simulink model "Zadanie_3_4_5"  (R2023b)
settings: Solver=VariableStepAuto  StartTime=0.0  StopTime=10  RelTol=1e-3
undefined symbols (not defined in the file or in its folder): m, R, v_phi, v_q, x0, y0
libraries: slpidlib x2
settings Model: Creator=student  LastModifiedBy=lukin

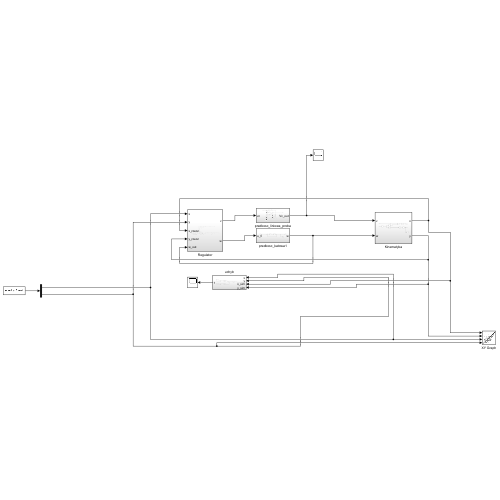
[thumbnail: Simulink's stored preview of the top-level diagram]
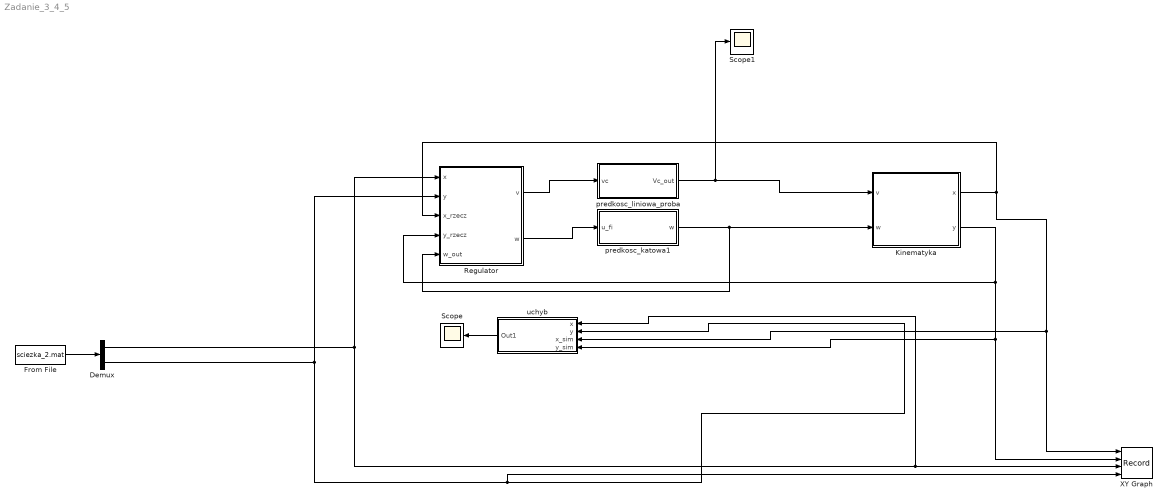
== system Zadanie_3_4_5 ==
  Demux : Demux  Outputs=2
  From File : FromFile  FileName=sciezka_2.mat  SampleTime=0
  Kinematyka : Subsystem
  Regulator : Subsystem
  Scope : Scope
  Scope1 : Scope
  XY Graph : Record  FileSettingsInternal="{\"entries\":[{\"content\":{\"excelSettings\":{\"content\":{},\"type\":\"Streamout.ExcelSettings\"}},\"type\":\"Streamout.FileSettingStorage\",\"uuid\":\"\"}],\"packageUris\":[\"http:\\/\\/schema.mathworks.com\\/mf0\\/streamout_blocks\\/R2020a\"],\"version\":\"1.0\"}"  Layout=[1 1]  SignalsInternal="{\"entries\":[{\"content\":{\"signals\":[{\"content\":{\"blockPath\":[],\"dimensions\":[1],\"domain\":\"\",\"lineColor\":\"#edb120\",\"plots\":[ 1 ],\"port\":1,\"sid\":[\"\"],\"signalID\":1,\"signalName\":\"Kinematyka:1\"},\"type\":\"RecordBlkView.Signal\",\"uuid\":\"\"},{\"content\":{\"blockPath\":[],\"dimensions\":[1],\"domain\":\"\",\"lineColor\":\"#7e2f8e\",\"plots\":[ 1 ],\"port\":2,\"sid\":[\"\"],\"signalID\":2,\"signalName\":\"Kinematyka:2\"},\"type\":\"RecordBlkView.Signal\",\"uuid\":\"\"},{\"content\":{\"blockPath\":[],\"dimensions\":[1],\"domain\":\"\",\"lineColor\":\"#7e2f8e\",\"plots\":[ 1 ],\"port\":3,\"sid\":[\"\"],\"signalID\":3,\"signalName\":\"Demux:1\"},\"type\":\"RecordBlkView.Signal\",\"uuid\":\"\"},{\"content\":{\"blockPath\":[],\"dimensions\":[1],\"domain\":\"\",\"lineColor\":\"#77ac30\",\"plots\":[ 1 ],\"port\":4,\"sid\":[\"\"],\"signalID\":4,\"signalName\":\"Demux:2\"},\"type\":\"RecordBlkView.Signal\",\"uuid\":\"\"}]},\"type\":\"RecordBlkView.InputSignals\",\"uuid\":\"\"}],\"packageUris\":[\"http:\\/\\/schema.mathworks.com\\/mf0\\/streamout_blocks\\/R2020a\"],\"version\":\"1.0\"}"  VisualizationBindings="{\"xyplotplugin\":{\"info\":[{\"series\":[{\"bindingParametersList\":[{\"parameter\":\"X-Axis\",\"signalID\":1,\"signalName\":\"Kinematyka:1\"},{\"parameter\":\"Y-Axis\",\"signalID\":2,\"signalName\":\"Kinematyka:2\"}],\"seriesID\":0},{\"bindingParametersList\":[{\"parameter\":\"X-Axis\",\"signalID\":3,\"signalName\":\"Demux:1\"},{\"parameter\":\"Y-Axis\",\"signalID\":4,\"signalName\":\"Demux:2\"}],\"seriesID\":1},{\"bindingParametersList\":[{\"parameter\":\"Y-Axis\",\"signalID\":4,\"signalName\":\"Demux:2\"}],\"seriesID\":2}],\"subplotID\":1}]}}"  CompatibilityTag=XY  st=-1
  predkosc_katowa1 : Subsystem
  predkosc_liniowa_proba : Subsystem
  uchyb : Subsystem
  wires:
  From File/1 -> Demux/1
  Demux/1 -> XY Graph/3, uchyb/1(x), Regulator/1(x)
  Demux/2 -> XY Graph/4, uchyb/2(y), Regulator/2(y)
  Kinematyka/1(x) -> XY Graph/1, uchyb/3(x_sim), Regulator/3(x_rzecz)
  Kinematyka/2(y) -> XY Graph/2, uchyb/4(y_sim), Regulator/4(y_rzecz)
  uchyb/1(Out1) -> Scope/1
  Regulator/2(w) -> predkosc_katowa1/1(u_fi)
  predkosc_katowa1/1(w) -> Regulator/5(w_out), Kinematyka/2(w)
  Regulator/1(v) -> predkosc_liniowa_proba/1(vc)
  predkosc_liniowa_proba/1(Vc_out) -> Kinematyka/1(v), Scope1/1

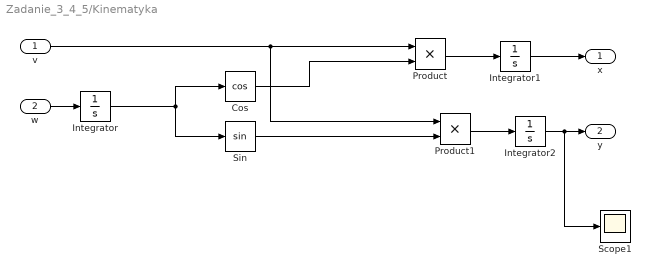
== system Zadanie_3_4_5/Kinematyka ==
  v : Inport
  w : Inport  Port=2
  Cos : Trigonometry  Operator=cos
  Integrator : Integrator  InitialCondition=v_phi
  Integrator1 : Integrator  InitialCondition=x0
  Integrator2 : Integrator  InitialCondition=y0
  Product : Product
  Product1 : Product
  Scope1 : Scope
  Sin : Trigonometry
  x : Outport
  y : Outport  Port=2
  wires:
  v/1 -> Product1/1, Product/1
  Cos/1 -> Product/2
  Product/1 -> Integrator1/1
  Integrator1/1 -> x/1
  Sin/1 -> Product1/2
  Product1/1 -> Integrator2/1
  Integrator2/1 -> Scope1/1, y/1
  w/1 -> Integrator/1
  Integrator/1 -> Cos/1, Sin/1

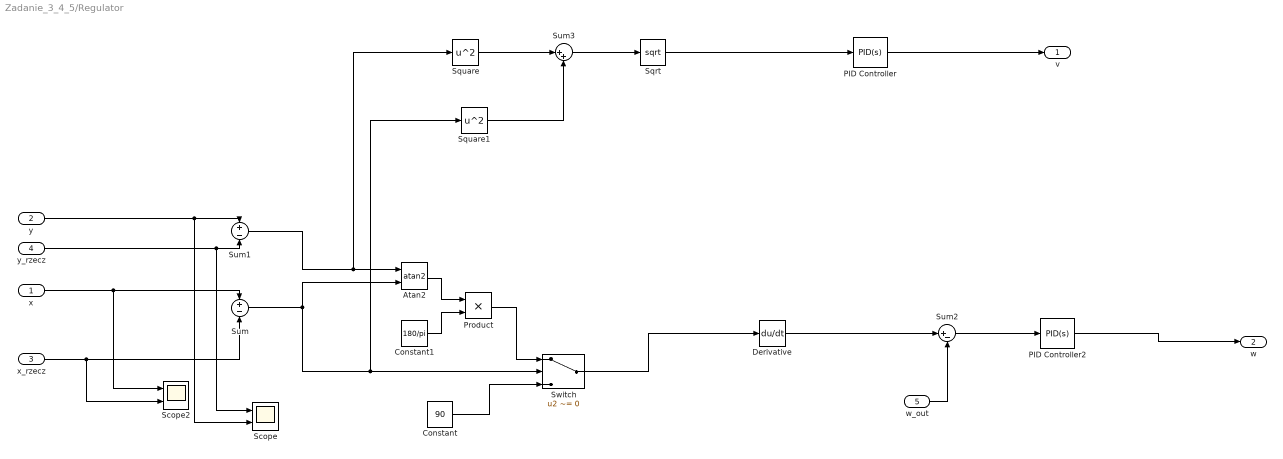
== system Zadanie_3_4_5/Regulator ==
  x : Inport
  y : Inport  Port=2
  x_rzecz : Inport  Port=3
  y_rzecz : Inport  Port=4
  w_out : Inport  Port=5
  Atan2 : Trigonometry  Operator=atan2  OutputSignalType=real
  Constant : Constant  Value=90
  Constant1 : Constant  Value=180/pi
  Derivative : Derivative
  PID Controller : slpidlib/PID Controller  Controller=PID  Form=Parallel  TimeDomain=Continuous-time  UseExternalTs=off  SampleTime=-1  IntegratorMethod=Forward Euler  FilterMethod=Forward Euler  ControllerParametersSource=internal  P=1.8  I=0  UseKiTs=off  D=0  N=100  UseFilter=on  TunerSelectOption=Transfer Function Based (PID Tuner App)  InitialConditionSource=internal  InitialConditionForIntegrator=0  InitialConditionForFilter=0  DifferentiatorICPrevScaledInput=0  ExternalReset=none  TrackingMode=off  Kt=1  LimitOutput=off  SatLimitsSource=internal  UpperSaturationLimit=inf  LowerSaturationLimit=-inf  LinearizeAsGain=on  AntiWindupMode=none  Kb=1  LimitIntegrator=off  UpperIntegratorSaturationLimit=inf  LowerIntegratorSaturationLimit=-inf  POutMin=[]  POutMax=[]  IOutMin=[]  IOutMax=[]  DOutMin=[]  DOutMax=[]  NOutMin=[]  NOutMax=[]  SumOutMin=[]  SumOutMax=[]  SaturationOutMin=[]  SaturationOutMax=[]  PParamMin=[]  PParamMax=[]  IParamMin=[]  IParamMax=[]  DParamMin=[]  DParamMax=[]  NParamMin=[]  NParamMax=[]  KbParamMin=[]  KbParamMax=[]  KtParamMin=[]  KtParamMax=[]  KbOutMin=[]  KbOutMax=[]  KtOutMin=[]  KtOutMax=[]  IntegratorOutMin=[]  IntegratorOutMax=[]  FilterOutMin=[]  FilterOutMax=[]  SumI1OutMin=[]  SumI1OutMax=[]  SumI2OutMin=[]  SumI2OutMax=[]  SumI3OutMin=[]  SumI3OutMax=[]  SumI4OutMin=[]  SumI4OutMax=[]  SumDOutMin=[]  SumDOutMax=[]  DifferentiatorOutMin=[]  DifferentiatorOutMax=[]  FilterDiffOutCoefMin=[]  FilterDiffOutCoefMax=[]  ReciprocalOutMin=[]  ReciprocalOutMax=[]  SumDenOutMin=[]  SumDenOutMax=[]  SumNumOutMin=[]  SumNumOutMax=[]  DivideOutMin=[]  DivideOutMax=[]  UdiffTsProdOutMin=[]  UdiffTsProdOutMax=[]  NTsProdOutMin=[]  NTsProdOutMax=[]  UintegralTsProdOutMin=[]  UintegralTsProdOutMax=[]  UngainTsProdOutMin=[]  UngainTsProdOutMax=[]  ClampingZeroOutDataTypeStr=Inherit: Inherit via back propagation  ClampingZeroOutMin=[]  ClampingZeroOutMax=[]  FilterDenConstantOutDataTypeStr=Inherit: Inherit via back propagation  FilterDenConstantOutMin=[]  FilterDenConstantOutMax=[]  PCopyOutDataTypeStr=Inherit: Inherit via back propagation  PCopyOutMin=[]  PCopyOutMax=[]  NCopyOutDataTypeStr=Inherit: Inherit via back propagation  NCopyOutMin=[]  NCopyOutMax=[]  IntegratorContinuousStateAttributes=''  IntegratorStateMustResolveToSignalObject=off  IntegratorRTWStateStorageClass=Auto  FilterContinuousStateAttributes=''  FilterStateMustResolveToSignalObject=off  FilterRTWStateStorageClass=Auto  ParallelPVariant=InternalParameters  IdealPVariant=Disabled  IVariant=InternalParameters  DVariant=InternalParameters  IntegratorVariant=Continuous  SatVariant=Disabled  AWVariant=Passthrough  PCopyVariant=Disabled  TRVariant=Disabled  FdbkBlocksVariant=Forward  IdealPFdbkVariant=Disabled  SatFdbkVariant=Disabled  DerivativeFilterVariant=ContFilter  NVariant=InternalParameters  NCopyVariant=Disabled  FilterICVariant=InternalICsFilter  IntegratorICVariant=InternalICs  ExternalResetVariant=Disabled  TRSumVariant=Passthrough  SumFdbkVariant=Disabled  SumVariant=Sum_PID  TsampFilterVariant=InternalTs  TsampNgainVariant=Passthrough  TsampIntegralVariant=Disabled_SignalSpec  ExternalSaturationOutDataTypeStr=Inherit: Same as second input
  PID Controller2 : slpidlib/PID Controller  Controller=PID  Form=Parallel  TimeDomain=Continuous-time  UseExternalTs=off  SampleTime=-1  IntegratorMethod=Forward Euler  FilterMethod=Forward Euler  ControllerParametersSource=internal  P=0.65  I=0.012  UseKiTs=off  D=0.012  N=100  UseFilter=on  TunerSelectOption=Transfer Function Based (PID Tuner App)  InitialConditionSource=internal  InitialConditionForIntegrator=0  InitialConditionForFilter=0  DifferentiatorICPrevScaledInput=0  ExternalReset=none  TrackingMode=off  Kt=1  LimitOutput=off  SatLimitsSource=internal  UpperSaturationLimit=inf  LowerSaturationLimit=-inf  LinearizeAsGain=on  AntiWindupMode=none  Kb=1  LimitIntegrator=off  UpperIntegratorSaturationLimit=inf  LowerIntegratorSaturationLimit=-inf  POutMin=[]  POutMax=[]  IOutMin=[]  IOutMax=[]  DOutMin=[]  DOutMax=[]  NOutMin=[]  NOutMax=[]  SumOutMin=[]  SumOutMax=[]  SaturationOutMin=[]  SaturationOutMax=[]  PParamMin=[]  PParamMax=[]  IParamMin=[]  IParamMax=[]  DParamMin=[]  DParamMax=[]  NParamMin=[]  NParamMax=[]  KbParamMin=[]  KbParamMax=[]  KtParamMin=[]  KtParamMax=[]  KbOutMin=[]  KbOutMax=[]  KtOutMin=[]  KtOutMax=[]  IntegratorOutMin=[]  IntegratorOutMax=[]  FilterOutMin=[]  FilterOutMax=[]  SumI1OutMin=[]  SumI1OutMax=[]  SumI2OutMin=[]  SumI2OutMax=[]  SumI3OutMin=[]  SumI3OutMax=[]  SumI4OutMin=[]  SumI4OutMax=[]  SumDOutMin=[]  SumDOutMax=[]  DifferentiatorOutMin=[]  DifferentiatorOutMax=[]  FilterDiffOutCoefMin=[]  FilterDiffOutCoefMax=[]  ReciprocalOutMin=[]  ReciprocalOutMax=[]  SumDenOutMin=[]  SumDenOutMax=[]  SumNumOutMin=[]  SumNumOutMax=[]  DivideOutMin=[]  DivideOutMax=[]  UdiffTsProdOutMin=[]  UdiffTsProdOutMax=[]  NTsProdOutMin=[]  NTsProdOutMax=[]  UintegralTsProdOutMin=[]  UintegralTsProdOutMax=[]  UngainTsProdOutMin=[]  UngainTsProdOutMax=[]  ClampingZeroOutDataTypeStr=Inherit: Inherit via back propagation  ClampingZeroOutMin=[]  ClampingZeroOutMax=[]  FilterDenConstantOutDataTypeStr=Inherit: Inherit via back propagation  FilterDenConstantOutMin=[]  FilterDenConstantOutMax=[]  PCopyOutDataTypeStr=Inherit: Inherit via back propagation  PCopyOutMin=[]  PCopyOutMax=[]  NCopyOutDataTypeStr=Inherit: Inherit via back propagation  NCopyOutMin=[]  NCopyOutMax=[]  IntegratorContinuousStateAttributes=''  IntegratorStateMustResolveToSignalObject=off  IntegratorRTWStateStorageClass=Auto  FilterContinuousStateAttributes=''  FilterStateMustResolveToSignalObject=off  FilterRTWStateStorageClass=Auto  ParallelPVariant=InternalParameters  IdealPVariant=Disabled  IVariant=InternalParameters  DVariant=InternalParameters  IntegratorVariant=Continuous  SatVariant=Disabled  AWVariant=Passthrough  PCopyVariant=Disabled  TRVariant=Disabled  FdbkBlocksVariant=Forward  IdealPFdbkVariant=Disabled  SatFdbkVariant=Disabled  DerivativeFilterVariant=ContFilter  NVariant=InternalParameters  NCopyVariant=Disabled  FilterICVariant=InternalICsFilter  IntegratorICVariant=InternalICs  ExternalResetVariant=Disabled  TRSumVariant=Passthrough  SumFdbkVariant=Disabled  SumVariant=Sum_PID  TsampFilterVariant=InternalTs  TsampNgainVariant=Passthrough  TsampIntegralVariant=Disabled_SignalSpec  ExternalSaturationOutDataTypeStr=Inherit: Same as second input
  Product : Product
  Scope : Scope  NumInputPorts=2
  Scope2 : Scope  NumInputPorts=2
  Sqrt : Sqrt
  Square : Math  Operator=square
  Square1 : Math  Operator=square
  Sum : Sum  Inputs=+-
  Sum1 : Sum  Inputs=+-
  Sum2 : Sum  Inputs=|+-
  Sum3 : Sum  Inputs=|++
  Switch : Switch  Criteria=u2 ~= 0  SaturateOnIntegerOverflow=off  InputSameDT=off
  v : Outport
  w : Outport  Port=2
  wires:
  x/1 -> Scope2/1, Sum/1
  Atan2/1 -> Product/1
  Constant1/1 -> Product/2
  x_rzecz/1 -> Scope2/2, Sum/2
  y_rzecz/1 -> Scope/1, Sum1/2
  Sum2/1 -> PID Controller2/1
  w_out/1 -> Sum2/2
  Switch/1 -> Derivative/1
  Constant/1 -> Switch/3
  Product/1 -> Switch/1
  Sum1/1 -> Square/1, Atan2/1
  Sum/1 -> Square1/1, Switch/2, Atan2/2
  Derivative/1 -> Sum2/1
  y/1 -> Scope/2, Sum1/1
  Square/1 -> Sum3/1
  Square1/1 -> Sum3/2
  Sum3/1 -> Sqrt/1
  PID Controller2/1 -> w/1
  Sqrt/1 -> PID Controller/1
  PID Controller/1 -> v/1

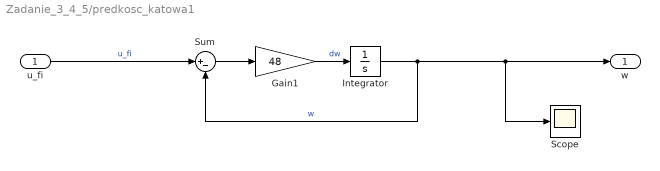
== system Zadanie_3_4_5/predkosc_katowa1 ==
  u_fi : Inport
  Gain1 : Gain  Gain=48
  Integrator : Integrator
  Scope : Scope
  Sum : Sum  Inputs=|+-
  w : Outport
  wires:
  Sum/1 -> Gain1/1
  u_fi/1 -> Sum/1  "u_fi"
  Integrator/1 -> w/1, Scope/1, Sum/2  "w"
  Gain1/1 -> Integrator/1  "dw"

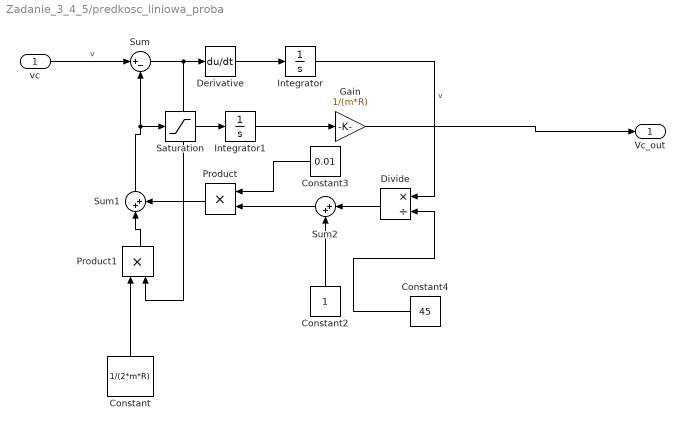
== system Zadanie_3_4_5/predkosc_liniowa_proba ==
  vc : Inport
  Constant : Constant  Value=1/(2*m*R)
  Constant2 : Constant
  Constant3 : Constant  Value=0.01
  Constant4 : Constant  Value=45
  Derivative : Derivative
  Divide : Product  Inputs=*/
  Gain : Gain  Gain=1/(m*R)
  Integrator : Integrator
  Integrator1 : Integrator  InitialCondition=v_q
  Product : Product
  Product1 : Product
  Saturation : Saturate  UpperLimit=10  LowerLimit=-10
  Sum : Sum  Inputs=|+-
  Sum1 : Sum  Inputs=|++
  Sum2 : Sum  Inputs=|++
  Vc_out : Outport
  wires:
  vc/1 -> Sum/1  "v"
  Sum/1 -> Product1/2, Derivative/1
  Integrator/1 -> Divide/1  "v"
  Constant4/1 -> Divide/2
  Divide/1 -> Sum2/1
  Constant2/1 -> Sum2/2
  Sum2/1 -> Product/2
  Constant3/1 -> Product/1
  Product/1 -> Sum1/2
  Sum1/1 -> Saturation/1, Sum/2
  Derivative/1 -> Integrator/1
  Integrator1/1 -> Gain/1
  Gain/1 -> Vc_out/1
  Constant/1 -> Product1/1
  Product1/1 -> Sum1/1
  Saturation/1 -> Integrator1/1

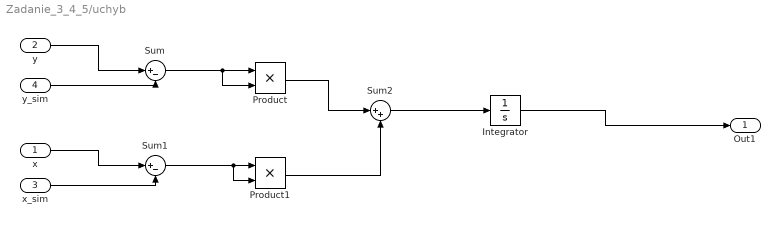
== system Zadanie_3_4_5/uchyb ==
  x : Inport
  y : Inport  Port=2
  x_sim : Inport  Port=3
  y_sim : Inport  Port=4
  Integrator : Integrator
  Product : Product
  Product1 : Product
  Sum : Sum  Inputs=|+-
  Sum1 : Sum  Inputs=|+-
  Sum2 : Sum  Inputs=|++
  Out1 : Outport
  wires:
  x/1 -> Sum1/1
  x_sim/1 -> Sum1/2
  y/1 -> Sum/1
  y_sim/1 -> Sum/2
  Sum/1 -> Product/2, Product/1
  Sum1/1 -> Product1/2, Product1/1
  Product/1 -> Sum2/1
  Sum2/1 -> Integrator/1
  Integrator/1 -> Out1/1
  Product1/1 -> Sum2/2
